simulink model "PID_2DOF"  (R2020b)
settings: Solver=ode4  StartTime=0  StopTime=20  FixedStep=0.01  RelTol=1e-1
settings Model: Creator=Admin  LastModifiedBy=Admin

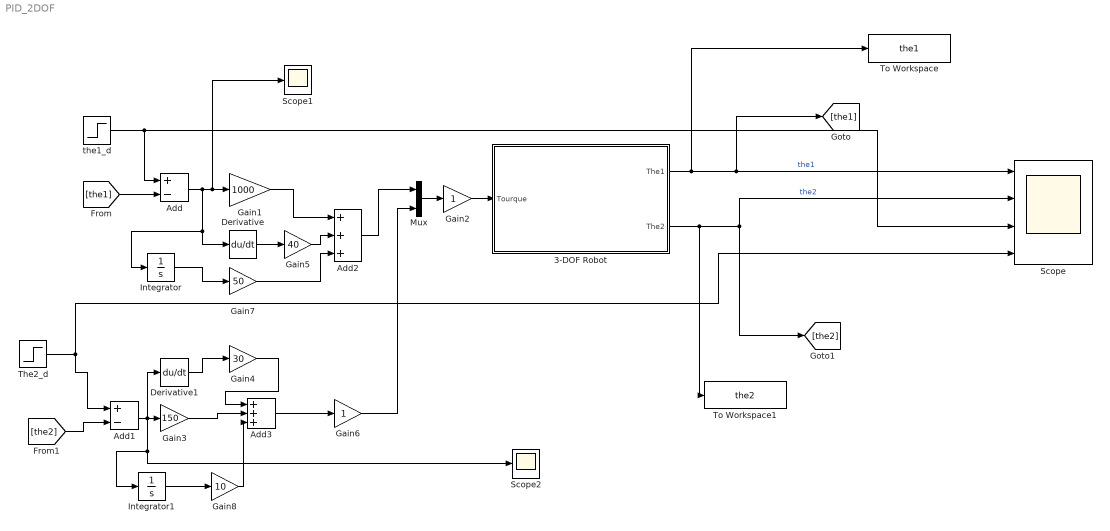
== system PID_2DOF ==
  3-DOF Robot : Subsystem
  Add : Sum  Inputs=+-
  Add1 : Sum  Inputs=+-
  Add2 : Sum  Inputs=+++
  Add3 : Sum  Inputs=+++
  Derivative : Derivative
  Derivative1 : Derivative
  Gain1 : Gain  Gain=1000
  Gain2 : Gain
  Gain3 : Gain  Gain=150
  Gain4 : Gain  Gain=30
  Gain5 : Gain  Gain=40
  Gain6 : Gain
  Gain7 : Gain  Gain=50
  Gain8 : Gain  Gain=10
  Integrator : Integrator
  Integrator1 : Integrator
  Mux : Mux  Inputs=2
  Scope : Scope  NumInputPorts=4
  Scope1 : Scope
  Scope2 : Scope
  The2_d : Step  Time=0  After=0  SampleTime=0
  To Workspace : ToWorkspace  VariableName=the1  SampleTime=-1
      settings: Save2DSignal=2-D array (concatenate along first dimension)
  To Workspace1 : ToWorkspace  VariableName=the2  SampleTime=-1
      settings: Save2DSignal=2-D array (concatenate along first dimension)
  the1_d : Step  Time=0  After=pi/2  SampleTime=0
  wires:
  3-DOF Robot/1(The1) -> [the1], Scope/1, To Workspace/1  "the1"
  3-DOF Robot/2(The2) -> To Workspace1/1, Scope/2, [the2]  "the2"
  the1_d/1 -> Add/1, Scope/3
  [the1] -> Add/2
  The2_d/1 -> Add1/1, Scope/4
  [the2] -> Add1/2
  Add/1 -> Integrator/1, Derivative/1, Scope1/1, Gain1/1
  Add1/1 -> Scope2/1, Integrator1/1, Derivative1/1, Gain3/1
  Gain3/1 -> Add3/2
  Mux/1 -> Gain2/1
  Gain2/1 -> 3-DOF Robot/1(Tourque)
  Gain1/1 -> Add2/1
  Derivative/1 -> Gain5/1
  Add2/1 -> Mux/1
  Derivative1/1 -> Gain4/1
  Add3/1 -> Gain6/1
  Gain4/1 -> Add3/1
  Gain5/1 -> Add2/2
  Gain6/1 -> Mux/2
  Integrator/1 -> Gain7/1
  Gain7/1 -> Add2/3
  Integrator1/1 -> Gain8/1
  Gain8/1 -> Add3/3

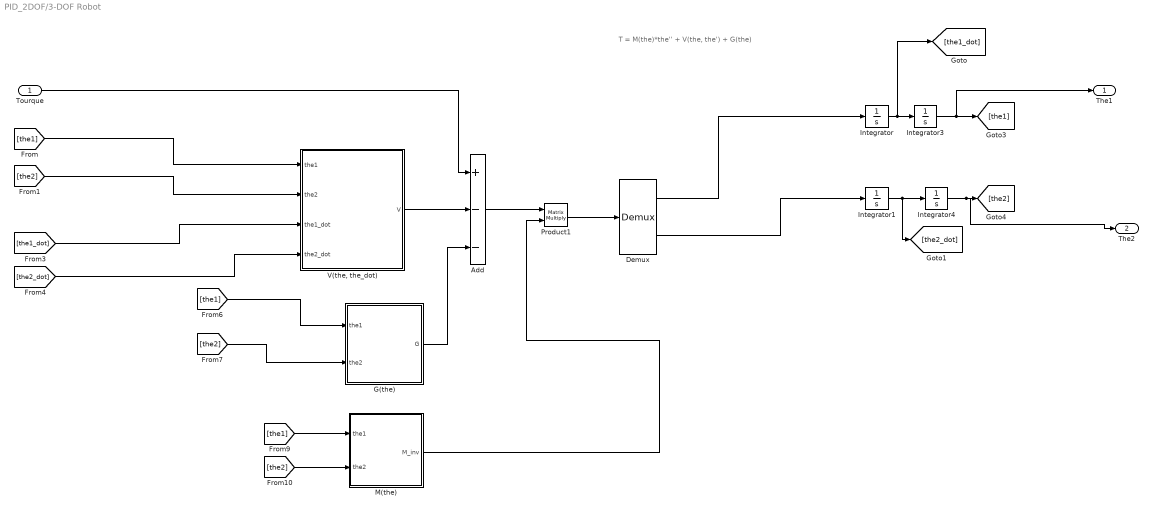
== system PID_2DOF/3-DOF Robot ==
  note: T = M(the)*the'' + V(the, the') + G(the)
  Tourque : Inport
  Add : Sum  Inputs=+--
  Demux : Demux  Outputs=2
      settings: DisplayOption=none
  G(the) : MATLAB Function  TreatAsAtomicUnit=on
  Integrator{,1,3..4} (4 alike) : Integrator
  M(the) : MATLAB Function  TreatAsAtomicUnit=on
  Product1 : Product  Multiplication=Matrix(*)
  "V(the, the_dot)" : MATLAB Function  TreatAsAtomicUnit=on
  The1 : Outport
  The2 : Outport  Port=2
  wires:
  Integrator4/1 -> The2/1, [the2]
  G(the)/1(G) -> Add/3
  [the1] -> G(the)/1(the1)
  Tourque/1 -> Add/1
  Integrator/1 -> [the1_dot], Integrator3/1
  Integrator1/1 -> [the2_dot], Integrator4/1
  Integrator3/1 -> The1/1, [the1]
  [the2] -> "V(the, the_dot)"/2(the2)
  [the2] -> M(the)/2(the2)
  [the1] -> "V(the, the_dot)"/1(the1)
  "V(the, the_dot)"/1(V) -> Add/2
  [the1] -> M(the)/1(the1)
  [the2] -> G(the)/2(the2)
  [the1_dot] -> "V(the, the_dot)"/3(the1_dot)
  [the2_dot] -> "V(the, the_dot)"/4(the2_dot)
  Add/1 -> Product1/1
  Demux/1 -> Integrator/1
  Demux/2 -> Integrator1/1
  Product1/1 -> Demux/1
  M(the)/1(M_inv) -> Product1/2

== matlab function PID_2DOF/3-DOF Robot/M(the) ==
  data: the1 input; M_inv output; the2 input
function M_inv = fcn(the1, the2)

% ROBOT parameters
m1 = 1;
m2 = 1;
m3 = 1;

l1 = 1;
l2 = 1;
l3 = 1;

J1 = 0.5;
J2 = 0.5;
J3 = 0.5;
g =9.81;


M = [ l2*l2*m2 + 2*l1*l2*m2*cos(the2)+ l1*l1*(m1+m2)    , l2*l2*m2 + l1*l2*m2*cos(the2) ;...
        l2*l2*m2 + l1*l2*m2*cos(the2) , l2*l2*m2];

M_inv = inv(M)

== matlab function PID_2DOF/3-DOF Robot/G(the) ==
  data: the1 input; G output; the2 input
function G = fcn(the1, the2)

% ROBOT parameters
m1 = 1;
m2 = 1;


l1 = 1;
l2 = 1;
l3 = 1;

J1 = 0.5;
J2 = 0.5;
J3 = 0.5;
g =9.81;

G = [m2*l2*g*cos(the1+the2) + (m1+m2)*l1*g*cos(the1);...
        m2*l2*g*cos(the1+the2)];

== matlab function PID_2DOF/3-DOF Robot/V(the, the_dot) ==
  data: the1 input; V output; the2 input; the1_dot input; the2_dot input
function V = fcn(the1, the2, the1_dot, the2_dot)

% ROBOT parameters
m1 = 1;
m2 = 1;
m3 = 1;

l1 = 1;
l2 = 1;
l3 = 1;

V = [-m2*l1*l2*sin(the2)*(the2_dot*the2_dot) - 2*m2*l1*l2*sin(the2)*the1_dot*the2_dot;...
        m2*l1*l2*sin(the2)*(the1_dot*the1_dot)];


V = V + [the1_dot; the2_dot];
